simulink model "openLoopBoiler"  (R2017a)
settings: Solver=FixedStepAuto  StartTime=0.0  StopTime=simTime  FixedStep=Dt  RelTol=1e-3  EnableMultiTasking=on
undefined symbols (not defined in the file or in its folder): D0, make, U0, Y0
settings Model: Creator=Pablo Diaz  LastModifiedBy=Felipe
settings OptimizationCC: LifeSpan=inf
settings DebuggingCC: SFUnexpectedBacktrackingDiag=warning  SFNoUnconditionalDefaultTransitionDiag=warning  SFExecutionAtInitializationDiag=none
settings GRTTargetCC: TargetLangStandard=C89/C90 (ANSI)
settings ConfigComp: CovMetricSettings=dw  CovHtmlReporting=on  CovSaveCumulativeToWorkspaceVar=on  CovSaveSingleToWorkspaceVar=on  CovExternalEMLEnable=off

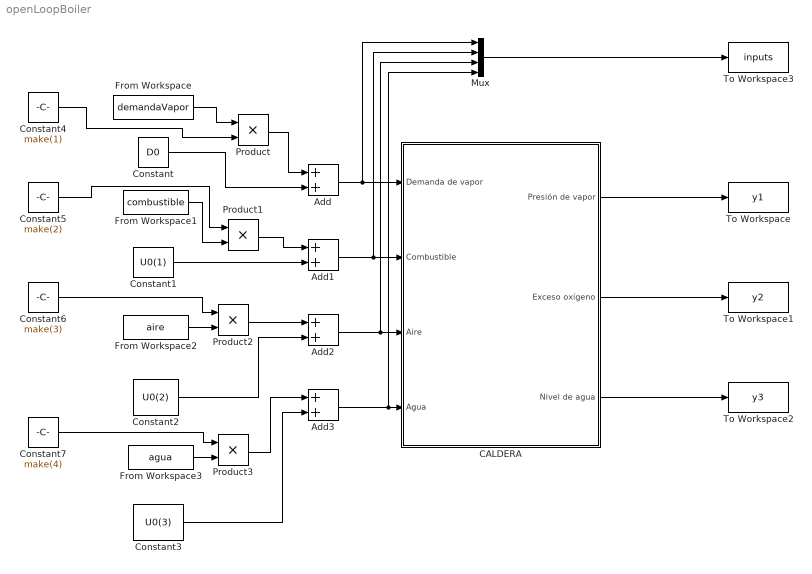
== system openLoopBoiler ==
  Add{,1..3} (4 alike) : Sum
  CALDERA : Subsystem
  Constant : Constant  Value=D0
  Constant1 : Constant  Value=U0(1)
  Constant2 : Constant  Value=U0(2)
  Constant3 : Constant  Value=U0(3)
  Constant4 : Constant  Value=make(1)
  Constant5 : Constant  Value=make(2)
  Constant6 : Constant  Value=make(3)
  Constant7 : Constant  Value=make(4)
  From Workspace : FromWorkspace  VariableName=demandaVapor  SampleTime=0
  From Workspace1 : FromWorkspace  VariableName=combustible  SampleTime=0
  From Workspace2 : FromWorkspace  VariableName=aire  SampleTime=0
  From Workspace3 : FromWorkspace  VariableName=agua  SampleTime=0
  Mux : Mux
  Product{,1..3} (4 alike) : Product
  To Workspace : ToWorkspace  VariableName=y1  SaveFormat=Structure With Time  SampleTime=-1
  To Workspace1 : ToWorkspace  VariableName=y2  SaveFormat=Structure With Time  SampleTime=-1
  To Workspace2 : ToWorkspace  VariableName=y3  SaveFormat=Structure With Time  SampleTime=-1
  To Workspace3 : ToWorkspace  VariableName=inputs  SaveFormat=Structure With Time  SampleTime=-1
  wires:
  CALDERA/2(Exceso oxígeno) -> To Workspace1/1
  CALDERA/3(Nivel de agua) -> To Workspace2/1
  From Workspace/1 -> Product/1
  Constant/1 -> Add/2
  From Workspace1/1 -> Product1/2
  Constant1/1 -> Add1/2
  From Workspace2/1 -> Product2/2
  Add2/1 -> Mux/3, CALDERA/3(Aire)
  Constant2/1 -> Add2/2
  From Workspace3/1 -> Product3/2
  Add3/1 -> Mux/4, CALDERA/4(Agua)
  Constant3/1 -> Add3/2
  Constant4/1 -> Product/2
  Product/1 -> Add/1
  Constant5/1 -> Product1/1
  Product1/1 -> Add1/1
  Constant6/1 -> Product2/1
  Product2/1 -> Add2/1
  Product3/1 -> Add3/1
  Constant7/1 -> Product3/1
  Add1/1 -> Mux/2, CALDERA/2(Combustible)
  Add/1 -> Mux/1, CALDERA/1(Demanda de vapor)
  Mux/1 -> To Workspace3/1
  CALDERA/1(Presión de vapor) -> To Workspace/1

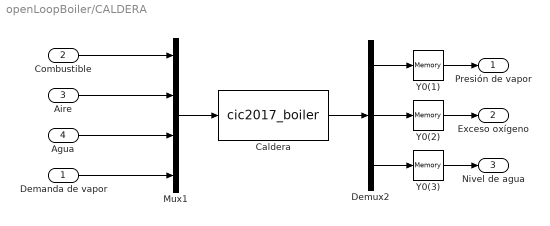
== system openLoopBoiler/CALDERA ==
  Demanda de vapor : Inport
  Combustible : Inport  Port=2
  Aire : Inport  Port=3
  Agua : Inport  Port=4
  Caldera : S-Function  FunctionName=cic2017_boiler  Parameters=Y0,[U0 D0]  SFunctionDeploymentMode=off  EnableBusSupport=off
  Demux2 : Demux  Outputs=3
  Mux1 : Mux
  Y0(1) : Memory  X0=Y0(1)
  Y0(2) : Memory  X0=Y0(2)
  Y0(3) : Memory  X0=Y0(3)
  Presión de vapor : Outport
  Exceso oxígeno : Outport  Port=2
  Nivel de agua : Outport  Port=3
  wires:
  Caldera/1 -> Demux2/1
  Aire/1 -> Mux1/2
  Agua/1 -> Mux1/3
  Demanda de vapor/1 -> Mux1/4
  Combustible/1 -> Mux1/1
  Mux1/1 -> Caldera/1
  Demux2/1 -> Y0(1)/1
  Demux2/2 -> Y0(2)/1
  Demux2/3 -> Y0(3)/1
  Y0(1)/1 -> Presión de vapor/1
  Y0(2)/1 -> Exceso oxígeno/1
  Y0(3)/1 -> Nivel de agua/1
